simulink model "CAT797_lateral_dynamics_differential_flatness_control_control_loop_2024"  (R2024a)
settings: Solver=FixedStepAuto  StartTime=0.0  StopTime=sim_t  FixedStep=0.01  RelTol=1e-3
PreLoadFcn:
  | clc; clear;
  | py_folder = 'G:\SIL_projects\carla_bridge';
  | if count(py.sys.path,py_folder) == 0
  |     insert(py.sys.path,int32(0),py_folder);
  | end
  | py.importlib.invalidate_caches();
  | mod = py.importlib.import_module('carla_bridge');
  | addpath("G:\Control_Research\Autonomy_Mining_Dump_Truck\src\plant_model\lib")
undefined symbols (not defined in the file or in its folder): Cf, Cr, Iz, k0, k1, ki, ky, Lf, Lr
libraries: simulink_extras x1
settings Model: DataDictionary=CAT_797F.sldd  Creator=marti343  LastModifiedBy=marti343
settings OptimizationCC: EnableMemcpy=off
settings HardwareCC: ProdBitPerChar=16  ProdBitPerInt=16  ProdBitPerPointer=32  ProdBitPerSizeT=32  ProdBitPerPtrDiffT=32  ProdLargestAtomicInteger=Integer  ProdLargestAtomicFloat=None  ProdWordSize=16  ProdHWDeviceType=Texas Instruments->C2000
settings RTWCC: GenerateReport=on  LaunchReport=on
settings CodeAppCC: ForceParamTrailComments=on  StateflowObjectComments=on  MATLABSourceComments=on
settings ConfigComp: CovBoundaryAbsTol=1.0e-5

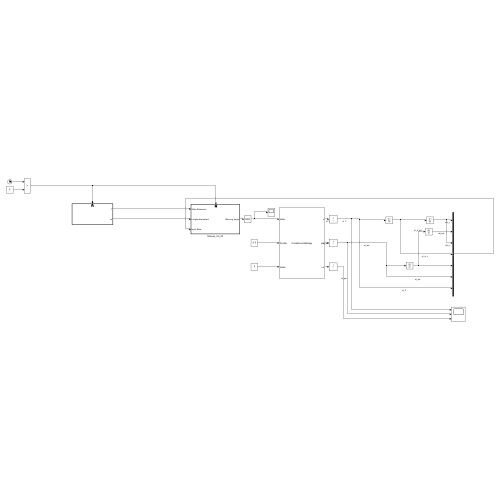
[thumbnail: Simulink's stored preview of the top-level diagram]
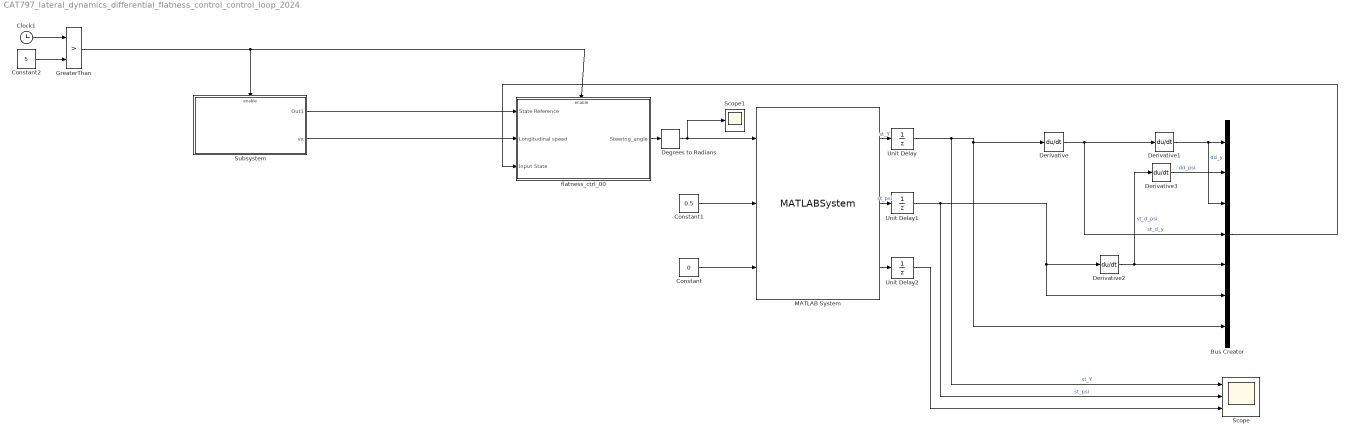
== system CAT797_lateral_dynamics_differential_flatness_control_control_loop_2024 ==
  Bus Creator : BusCreator  Inputs=7
  Clock1 : Clock
  Constant : Constant  Value=0
  Constant1 : Constant  Value=0.5
  Constant2 : Constant  Value=5
  Degrees to Radians : simulink_extras/Transformations/Degrees to Radians
  Derivative{,1..3} (4 alike) : Derivative
  GreaterThan : RelationalOperator  Operator=>  OutDataTypeStr=boolean  RndMeth=Simplest  InputSameDT=off
  MATLAB System : MATLABSystem  System=CarlaSimulinkBridge  PythonFolder=G:\Control_Research\Autonomy_Mining_Dump_Truck\src\plant_model  SimulateUsing=Interpreted execution
      mask Type: CarlaSimulinkBridge
      mask Display:
      | disp('CarlaSimulinkBridge');
      | port_label('input',1,'steer');
      | port_label('input',2,'throttle');
      | port_label('input',3,'brake');
      | port_label('output',1,'y');
      | port_label('output',2,'psi');
      | port_label('output',3,'vx');
  Scope : Scope  NumInputPorts=3
  Scope1 : Scope
  Subsystem : Subsystem
  Unit Delay : UnitDelay  SampleTime=0.05  HasFrameUpgradeWarning=on
  Unit Delay1 : UnitDelay  SampleTime=0.05  HasFrameUpgradeWarning=on
  Unit Delay2 : UnitDelay  SampleTime=0.05  HasFrameUpgradeWarning=on
  flatness_ctrl_00 : Subsystem
  wires:
  Derivative1/1 -> Bus Creator/3, Bus Creator/1  "dd_y"
  Derivative/1 -> Derivative1/1, Bus Creator/4  "st_d_y"
  Derivative3/1 -> Bus Creator/2  "dd_psi"
  MATLAB System/2 -> Unit Delay1/1  "st_psi"
  MATLAB System/1 -> Unit Delay/1  "st_Y"
  Derivative2/1 -> Bus Creator/5, Derivative3/1  "st_d_psi"
  Bus Creator/1 -> flatness_ctrl_00/3(Input State)
  flatness_ctrl_00/1(Steering_angle) -> Degrees to Radians/1
  MATLAB System/3 -> Unit Delay2/1
  Constant/1 -> MATLAB System/3
  Constant1/1 -> MATLAB System/2
  Unit Delay/1 -> Scope/1, Bus Creator/7, Derivative/1  "st_Y"
  Unit Delay1/1 -> Scope/2, Bus Creator/6, Derivative2/1  "st_psi"
  Unit Delay2/1 -> Scope/3
  Clock1/1 -> GreaterThan/1
  Constant2/1 -> GreaterThan/2
  GreaterThan/1 -> Subsystem/Enable, flatness_ctrl_00/Enable
  Subsystem/1(Out1) -> flatness_ctrl_00/1(State Reference)
  Subsystem/2(vx) -> flatness_ctrl_00/2(Longitudinal speed)
  Degrees to Radians/1 -> Scope1/1, MATLAB System/1

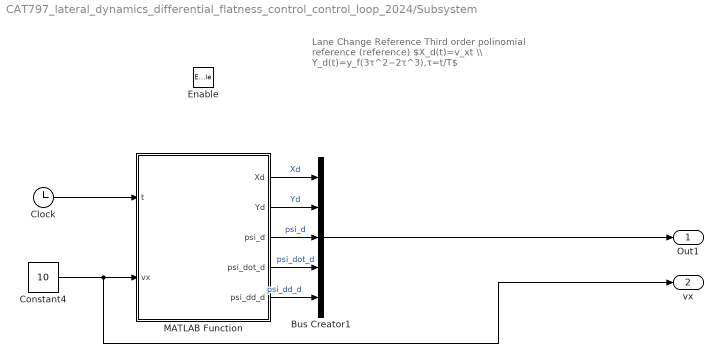
== system CAT797_lateral_dynamics_differential_flatness_control_control_loop_2024/Subsystem ==
  note: Lane Change Reference
      |
      | Third order polinomial reference (reference)
      | $X_d​(t)=v_x​t \\ Y_d(t)=y_f(3τ^2−2τ^3),τ=t/T$
  Enable : EnablePort
  Bus Creator1 : BusCreator  Inputs=5
  Clock : Clock
  Constant4 : Constant  Value=10
  MATLAB Function : MATLAB Function  TreatAsAtomicUnit=on
  Out1 : Outport
  vx : Outport  Port=2
  wires:
  MATLAB Function/4(psi_dot_d) -> Bus Creator1/4  "psi_dot_d"
  MATLAB Function/2(Yd) -> Bus Creator1/2  "Yd"
  Constant4/1 -> vx/1, MATLAB Function/2(vx)
  MATLAB Function/5(psi_dd_d) -> Bus Creator1/5  "psi_dd_d"
  MATLAB Function/1(Xd) -> Bus Creator1/1  "Xd"
  Clock/1 -> MATLAB Function/1(t)
  MATLAB Function/3(psi_d) -> Bus Creator1/3  "psi_d"
  Bus Creator1/1 -> Out1/1

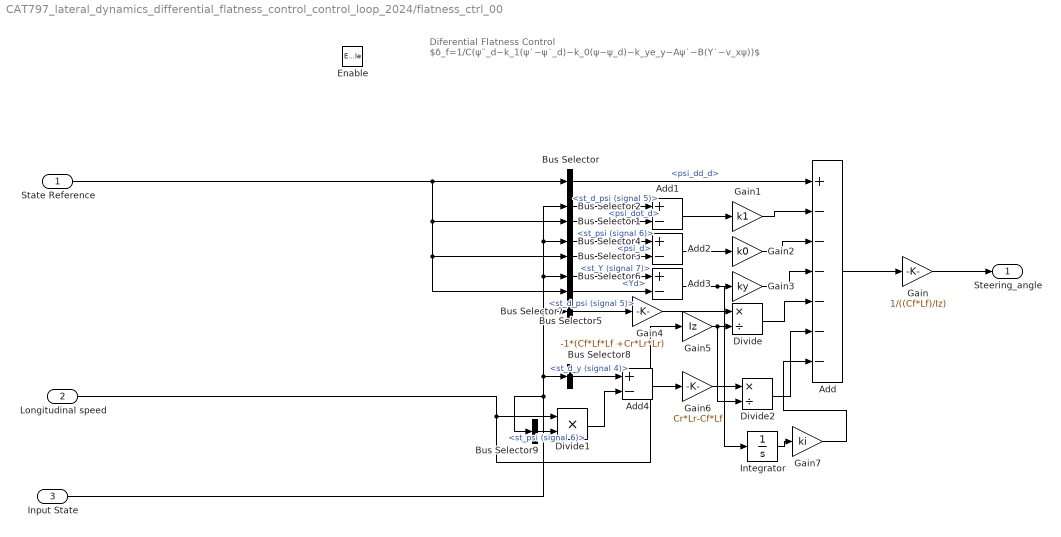
== system CAT797_lateral_dynamics_differential_flatness_control_control_loop_2024/flatness_ctrl_00 ==
  note: Diferential Flatness Control
      |
      | $δ_f​=1/C​(ψ¨_d​−k_1​(ψ˙​−ψ˙​_d​)−k_0​(ψ−ψ_d​)−k_y​e_y​−Aψ˙​−B(Y˙−v_x​ψ))$
  State Reference : Inport
  Longitudinal speed : Inport  Port=2
  Input State : Inport  Port=3
  Enable : EnablePort
  Add : Sum  Inputs=+------
  Add{1..4} (4 alike) : Sum  Inputs=+-
  Bus Selector : BusSelector  OutputSignals=psi_dd_d
  Bus Selector1 : BusSelector  OutputSignals=psi_dot_d
  Bus Selector2 : BusSelector  OutputSignals=st_d_psi (signal 5)
  Bus Selector3 : BusSelector  OutputSignals=psi_d
  Bus Selector4 : BusSelector  OutputSignals=st_psi (signal 6)
  Bus Selector5 : BusSelector  OutputSignals=Yd
  Bus Selector6 : BusSelector  OutputSignals=st_Y (signal 7)
  Bus Selector7 : BusSelector  OutputSignals=st_d_psi (signal 5)
  Bus Selector8 : BusSelector  OutputSignals=st_d_y (signal 4)
  Bus Selector9 : BusSelector  OutputSignals=st_psi (signal 6)
  Divide : Product  Inputs=*/
  Divide1 : Product  Inputs=**
  Divide2 : Product  Inputs=*/
  Gain : Gain  Gain=1/((Cf*Lf)/Iz)
  Gain1 : Gain  Gain=k1
  Gain2 : Gain  Gain=k0
  Gain3 : Gain  Gain=ky
  Gain4 : Gain  Gain=-1*(Cf*Lf*Lf +Cr*Lr*Lr)
  Gain5 : Gain  Gain=Iz
  Gain6 : Gain  Gain=Cr*Lr-Cf*Lf
  Gain7 : Gain  Gain=ki
  Integrator : Integrator
  Steering_angle : Outport
  wires:
  Add/1 -> Gain/1
  Gain2/1 -> Add/3
  Add3/1 -> Integrator/1, Gain3/1
  Divide1/1 -> Add4/2
  Divide2/1 -> Add/6
  Input State/1 -> Bus Selector2/1, Bus Selector4/1, Bus Selector6/1, Bus Selector7/1, Bus Selector8/1, Bus Selector9/1
  State Reference/1 -> Bus Selector5/1, Bus Selector3/1, Bus Selector1/1, Bus Selector/1
  Gain5/1 -> Divide2/2, Divide/2
  Bus Selector7/1 -> Gain4/1  "<st_d_psi (signal 5)>"
  Bus Selector4/1 -> Add2/1  "<st_psi (signal 6)>"
  Bus Selector1/1 -> Add1/2  "<psi_dot_d>"
  Bus Selector5/1 -> Add3/2  "<Yd>"
  Bus Selector9/1 -> Divide1/2  "<st_psi (signal 6)>"
  Gain7/1 -> Add/7
  Gain1/1 -> Add/2
  Add2/1 -> Gain2/1
  Gain/1 -> Steering_angle/1
  Gain3/1 -> Add/4
  Bus Selector6/1 -> Add3/1  "<st_Y (signal 7)>"
  Add1/1 -> Gain1/1
  Bus Selector3/1 -> Add2/2  "<psi_d>"
  Longitudinal speed/1 -> Gain5/1, Divide1/1
  Integrator/1 -> Gain7/1
  Bus Selector/1 -> Add/1  "<psi_dd_d>"
  Bus Selector2/1 -> Add1/1  "<st_d_psi (signal 5)>"
  Add4/1 -> Gain6/1
  Bus Selector8/1 -> Add4/1  "<st_d_y (signal 4)>"
  Divide/1 -> Add/5
  Gain6/1 -> Divide2/1
  Gain4/1 -> Divide/1

== matlab function CAT797_lateral_dynamics_differential_flatness_control_control_loop_2024/Subsystem/MATLAB Function ==
  data: t input; Xd output; vx input; Yd output; psi_d output; psi_dot_d output; psi_dd_d output
function [Xd, Yd, psi_d, psi_dot_d, psi_dd_d] = lane_change(t, vx)

% PARAMETERS (tune these)
T  = 10;       % duration [s]
yf = 3.5;      % lateral shift [m]

% Normalize time
tau = t / T;

% Clamp tau between 0 and 1
if tau > 1
    tau = 1;
end
if tau < 0
    tau = 0;
end

% =========================
% POSITION
% =========================
Xd = vx * t;
Yd = yf * (3*tau^2 - 2*tau^3);

% =========================
% FIRST DERIVATIVE
% =========================
Xd_dot = vx;
Yd_dot = yf * (6*tau/T - 6*tau^2/T);

% =========================
% SECOND DERIVATIVE
% =========================
Xd_ddot = 0;
Yd_ddot = yf * (6/T^2 - 12*tau/T^2);

% =========================
% HEADING
% =========================
psi_d = atan2(Yd_dot, Xd_dot);

% =========================
% YAW RATE
% =========================
psi_dot_d = (Xd_dot * Yd_ddot - Yd_dot * Xd_ddot) / ...
            (Xd_dot^2 + Yd_dot^2);

% =========================
% YAW ACCELERATION (optional)
% =========================
% Numerical approximation (simple)
dt = 1e-3;

tau2 = (t+dt)/T;
if tau2 > 1
    tau2 = 1;
end

Yd_dot_2 = yf * (6*tau2/T - 6*tau2^2/T);
psi_d_2 = atan2(Yd_dot_2, vx);

psi_dd_d = (psi_d_2 - psi_d) / dt;

end
